simulink model "ctrl_student_HIL"  (R2015a)
settings: Solver=ode4  StartTime=0.0  StopTime=inf  FixedStep=0.01  RelTol=1e-3
(part 2 of 2)

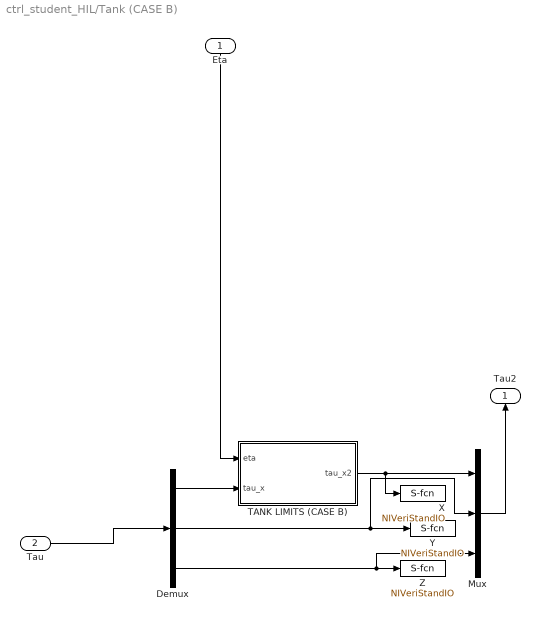
== system ctrl_student_HIL/Tank (CASE B) ==
  Eta : Inport
  Tau : Inport  Port=2
  Demux : Demux  Outputs=3
  Mux : Mux  Inputs=3
  TANK LIMITS (CASE B) : Subsystem
  X : S-Function  Priority=3  FunctionName=NIVeriStandIO  Parameters=width dtype portnum stime stype btype  mask(NI VeriStand Outport){portnum=3, width=-1, stime=-1, dtype=auto, stype=auto, btype=0}
      mask prompts: portnum "Port number:"; width "Port dimensions (-1 for dynamically sized):"; stime "Sample time (-1 for inherited):"; dtype "Data type:"; stype "Signal type:"; btype "Block type:"
      mask help: Use this outport on any level of nested subsystems to allow NI VeriStand software to map signals to it.
      mask init:
      | NIVeriStandIO_init;
      settings: CopyFcn=NIVeriStand_MDL_functions('', 'IO_copy');  DeleteFcn=NIVeriStand_MDL_functions('', 'IO_delete');  MoveFcn=set_param(gcb, 'Mask', 'on');
      mask Callback portnum: NIVeriStand_MDL_functions('', 'IO_setportnum');
      mask TypeOptions dtype: auto | double | single | int8 | uint8 | int16 | uint16 | int32 | uint32 | boolean
      mask Callback dtype: NIVeriStand_MDL_functions('', 'IO_booleansignal');
      mask TypeOptions stype: auto | real | complex
      mask Display:
      | patch([-x x], [-y y], [.90980 .81960 .32156]);
      | plot([xrad -x x xrad], [yrad -y y yrad]);
      | fprintf('NI Out%d', portnum);
  Y : S-Function  Priority=7  FunctionName=NIVeriStandIO  Parameters=width dtype portnum stime stype btype  mask(NI VeriStand Outport){portnum=7, width=-1, stime=-1, dtype=auto, stype=auto, btype=0}
      mask prompts: portnum "Port number:"; width "Port dimensions (-1 for dynamically sized):"; stime "Sample time (-1 for inherited):"; dtype "Data type:"; stype "Signal type:"; btype "Block type:"
      mask help: Use this outport on any level of nested subsystems to allow NI VeriStand software to map signals to it.
      mask init:
      | NIVeriStandIO_init;
      settings: CopyFcn=NIVeriStand_MDL_functions('', 'IO_copy');  DeleteFcn=NIVeriStand_MDL_functions('', 'IO_delete');  MoveFcn=set_param(gcb, 'Mask', 'on');
      mask Callback portnum: NIVeriStand_MDL_functions('', 'IO_setportnum');
      mask TypeOptions dtype: auto | double | single | int8 | uint8 | int16 | uint16 | int32 | uint32 | boolean
      mask Callback dtype: NIVeriStand_MDL_functions('', 'IO_booleansignal');
      mask TypeOptions stype: auto | real | complex
      mask Display:
      | patch([-x x], [-y y], [.90980 .81960 .32156]);
      | plot([xrad -x x xrad], [yrad -y y yrad]);
      | fprintf('NI Out%d', portnum);
  Z : S-Function  Priority=8  FunctionName=NIVeriStandIO  Parameters=width dtype portnum stime stype btype  mask(NI VeriStand Outport){portnum=8, width=-1, stime=-1, dtype=auto, stype=auto, btype=0}
      mask prompts: portnum "Port number:"; width "Port dimensions (-1 for dynamically sized):"; stime "Sample time (-1 for inherited):"; dtype "Data type:"; stype "Signal type:"; btype "Block type:"
      mask help: Use this outport on any level of nested subsystems to allow NI VeriStand software to map signals to it.
      mask init:
      | NIVeriStandIO_init;
      settings: CopyFcn=NIVeriStand_MDL_functions('', 'IO_copy');  DeleteFcn=NIVeriStand_MDL_functions('', 'IO_delete');  MoveFcn=set_param(gcb, 'Mask', 'on');
      mask Callback portnum: NIVeriStand_MDL_functions('', 'IO_setportnum');
      mask TypeOptions dtype: auto | double | single | int8 | uint8 | int16 | uint16 | int32 | uint32 | boolean
      mask Callback dtype: NIVeriStand_MDL_functions('', 'IO_booleansignal');
      mask TypeOptions stype: auto | real | complex
      mask Display:
      | patch([-x x], [-y y], [.90980 .81960 .32156]);
      | plot([xrad -x x xrad], [yrad -y y yrad]);
      | fprintf('NI Out%d', portnum);
  Tau2 : Outport
  wires:
  Mux/1 -> Tau2/1
  Tau/1 -> Demux/1
  TANK LIMITS (CASE B)/1(tau_x2) -> X/1, Mux/1
  Demux/1 -> TANK LIMITS (CASE B)/2(tau_x)
  Demux/2 -> Y/1, Mux/2
  Demux/3 -> Mux/3, Z/1
  Eta/1 -> TANK LIMITS (CASE B)/1(eta)

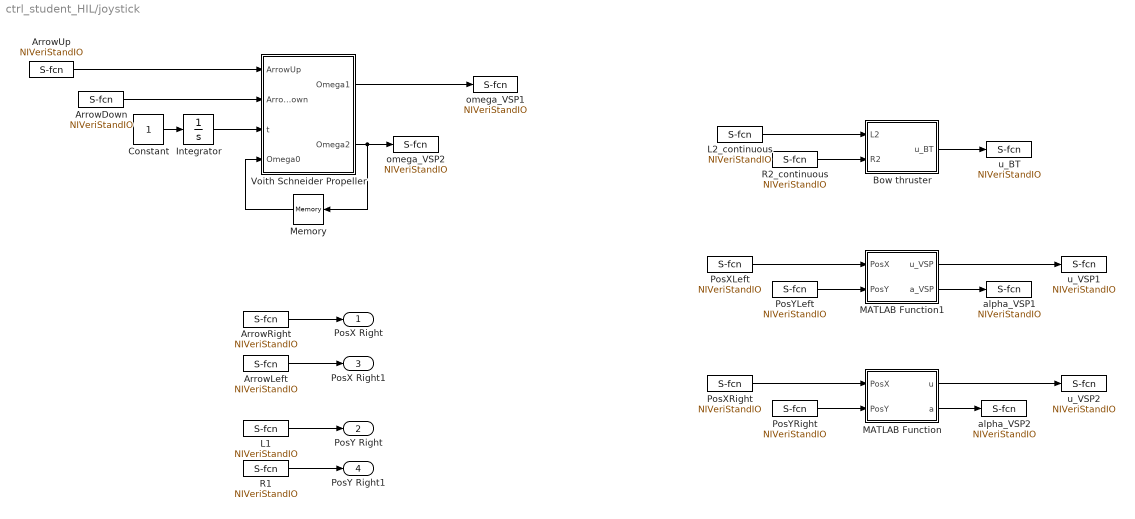
== system ctrl_student_HIL/joystick ==
  ArrowDown : S-Function  Priority=9  FunctionName=NIVeriStandIO  Parameters=width dtype portnum stime stype btype  mask(NI VeriStand Inport){portnum=9, width=-1, stime=-1, dtype=auto, stype=auto, btype=1}
      mask prompts: portnum "Port number:"; width "Port dimensions (-1 for dynamically sized):"; stime "Sample time (-1 for inherited):"; dtype "Data type:"; stype "Signal type:"; btype "Block type:"
      mask help: Use this inport on any level of nested subsystems to allow NI VeriStand software to map signals to it.
      mask init:
      | NIVeriStandIO_init;
      settings: CopyFcn=NIVeriStand_MDL_functions('', 'IO_copy');  DeleteFcn=NIVeriStand_MDL_functions('', 'IO_delete');  MoveFcn=set_param(gcb, 'Mask', 'on');
      mask Callback portnum: NIVeriStand_MDL_functions('', 'IO_setportnum');
      mask TypeOptions dtype: auto | double | single | int8 | uint8 | int16 | uint16 | int32 | uint32 | boolean
      mask Callback dtype: NIVeriStand_MDL_functions('', 'IO_booleansignal');
      mask TypeOptions stype: auto | real | complex
      mask Display:
      | patch([-x x], [-y y], [.90980 .81960 .32156]);
      | plot([xrad -x x xrad], [yrad -y y yrad]);
      | fprintf('NI In%d', portnum);
  ArrowLeft : S-Function  Priority=11  FunctionName=NIVeriStandIO  Parameters=width dtype portnum stime stype btype  mask(NI VeriStand Inport){portnum=11, width=-1, stime=-1, dtype=auto, stype=auto, btype=1}
      mask prompts: portnum "Port number:"; width "Port dimensions (-1 for dynamically sized):"; stime "Sample time (-1 for inherited):"; dtype "Data type:"; stype "Signal type:"; btype "Block type:"
      mask help: Use this inport on any level of nested subsystems to allow NI VeriStand software to map signals to it.
      mask init:
      | NIVeriStandIO_init;
      settings: CopyFcn=NIVeriStand_MDL_functions('', 'IO_copy');  DeleteFcn=NIVeriStand_MDL_functions('', 'IO_delete');  MoveFcn=set_param(gcb, 'Mask', 'on');
      mask Callback portnum: NIVeriStand_MDL_functions('', 'IO_setportnum');
      mask TypeOptions dtype: auto | double | single | int8 | uint8 | int16 | uint16 | int32 | uint32 | boolean
      mask Callback dtype: NIVeriStand_MDL_functions('', 'IO_booleansignal');
      mask TypeOptions stype: auto | real | complex
      mask Display:
      | patch([-x x], [-y y], [.90980 .81960 .32156]);
      | plot([xrad -x x xrad], [yrad -y y yrad]);
      | fprintf('NI In%d', portnum);
  ArrowRight : S-Function  Priority=12  FunctionName=NIVeriStandIO  Parameters=width dtype portnum stime stype btype  mask(NI VeriStand Inport){portnum=12, width=-1, stime=-1, dtype=auto, stype=auto, btype=1}
      mask prompts: portnum "Port number:"; width "Port dimensions (-1 for dynamically sized):"; stime "Sample time (-1 for inherited):"; dtype "Data type:"; stype "Signal type:"; btype "Block type:"
      mask help: Use this inport on any level of nested subsystems to allow NI VeriStand software to map signals to it.
      mask init:
      | NIVeriStandIO_init;
      settings: CopyFcn=NIVeriStand_MDL_functions('', 'IO_copy');  DeleteFcn=NIVeriStand_MDL_functions('', 'IO_delete');  MoveFcn=set_param(gcb, 'Mask', 'on');
      mask Callback portnum: NIVeriStand_MDL_functions('', 'IO_setportnum');
      mask TypeOptions dtype: auto | double | single | int8 | uint8 | int16 | uint16 | int32 | uint32 | boolean
      mask Callback dtype: NIVeriStand_MDL_functions('', 'IO_booleansignal');
      mask TypeOptions stype: auto | real | complex
      mask Display:
      | patch([-x x], [-y y], [.90980 .81960 .32156]);
      | plot([xrad -x x xrad], [yrad -y y yrad]);
      | fprintf('NI In%d', portnum);
  ArrowUp : S-Function  Priority=10  FunctionName=NIVeriStandIO  Parameters=width dtype portnum stime stype btype  mask(NI VeriStand Inport){portnum=10, width=-1, stime=-1, dtype=auto, stype=auto, btype=1}
      mask prompts: portnum "Port number:"; width "Port dimensions (-1 for dynamically sized):"; stime "Sample time (-1 for inherited):"; dtype "Data type:"; stype "Signal type:"; btype "Block type:"
      mask help: Use this inport on any level of nested subsystems to allow NI VeriStand software to map signals to it.
      mask init:
      | NIVeriStandIO_init;
      settings: CopyFcn=NIVeriStand_MDL_functions('', 'IO_copy');  DeleteFcn=NIVeriStand_MDL_functions('', 'IO_delete');  MoveFcn=set_param(gcb, 'Mask', 'on');
      mask Callback portnum: NIVeriStand_MDL_functions('', 'IO_setportnum');
      mask TypeOptions dtype: auto | double | single | int8 | uint8 | int16 | uint16 | int32 | uint32 | boolean
      mask Callback dtype: NIVeriStand_MDL_functions('', 'IO_booleansignal');
      mask TypeOptions stype: auto | real | complex
      mask Display:
      | patch([-x x], [-y y], [.90980 .81960 .32156]);
      | plot([xrad -x x xrad], [yrad -y y yrad]);
      | fprintf('NI In%d', portnum);
  Bow thruster : MATLAB Function  TreatAsAtomicUnit=on
  Constant : Constant
  Integrator : Integrator
  L1 : S-Function  Priority=7  FunctionName=NIVeriStandIO  Parameters=width dtype portnum stime stype btype  mask(NI VeriStand Inport){portnum=7, width=-1, stime=-1, dtype=auto, stype=auto, btype=1}
      mask prompts: portnum "Port number:"; width "Port dimensions (-1 for dynamically sized):"; stime "Sample time (-1 for inherited):"; dtype "Data type:"; stype "Signal type:"; btype "Block type:"
      mask help: Use this inport on any level of nested subsystems to allow NI VeriStand software to map signals to it.
      mask init:
      | NIVeriStandIO_init;
      settings: CopyFcn=NIVeriStand_MDL_functions('', 'IO_copy');  DeleteFcn=NIVeriStand_MDL_functions('', 'IO_delete');  MoveFcn=set_param(gcb, 'Mask', 'on');
      mask Callback portnum: NIVeriStand_MDL_functions('', 'IO_setportnum');
      mask TypeOptions dtype: auto | double | single | int8 | uint8 | int16 | uint16 | int32 | uint32 | boolean
      mask Callback dtype: NIVeriStand_MDL_functions('', 'IO_booleansignal');
      mask TypeOptions stype: auto | real | complex
      mask Display:
      | patch([-x x], [-y y], [.90980 .81960 .32156]);
      | plot([xrad -x x xrad], [yrad -y y yrad]);
      | fprintf('NI In%d', portnum);
  L2_continuous : S-Function  Priority=1  FunctionName=NIVeriStandIO  Parameters=width dtype portnum stime stype btype  mask(NI VeriStand Inport){portnum=1, width=-1, stime=-1, dtype=auto, stype=auto, btype=1}
      mask prompts: portnum "Port number:"; width "Port dimensions (-1 for dynamically sized):"; stime "Sample time (-1 for inherited):"; dtype "Data type:"; stype "Signal type:"; btype "Block type:"
      mask help: Use this inport on any level of nested subsystems to allow NI VeriStand software to map signals to it.
      mask init:
      | NIVeriStandIO_init;
      settings: CopyFcn=NIVeriStand_MDL_functions('', 'IO_copy');  DeleteFcn=NIVeriStand_MDL_functions('', 'IO_delete');  MoveFcn=set_param(gcb, 'Mask', 'on');
      mask Callback portnum: NIVeriStand_MDL_functions('', 'IO_setportnum');
      mask TypeOptions dtype: auto | double | single | int8 | uint8 | int16 | uint16 | int32 | uint32 | boolean
      mask Callback dtype: NIVeriStand_MDL_functions('', 'IO_booleansignal');
      mask TypeOptions stype: auto | real | complex
      mask Display:
      | patch([-x x], [-y y], [.90980 .81960 .32156]);
      | plot([xrad -x x xrad], [yrad -y y yrad]);
      | fprintf('NI In%d', portnum);
  MATLAB Function : MATLAB Function  TreatAsAtomicUnit=on
  MATLAB Function1 : MATLAB Function  TreatAsAtomicUnit=on
  Memory : Memory
  PosXLeft : S-Function  Priority=5  FunctionName=NIVeriStandIO  Parameters=width dtype portnum stime stype btype  mask(NI VeriStand Inport){portnum=5, width=-1, stime=-1, dtype=auto, stype=auto, btype=1}
      mask prompts: portnum "Port number:"; width "Port dimensions (-1 for dynamically sized):"; stime "Sample time (-1 for inherited):"; dtype "Data type:"; stype "Signal type:"; btype "Block type:"
      mask help: Use this inport on any level of nested subsystems to allow NI VeriStand software to map signals to it.
      mask init:
      | NIVeriStandIO_init;
      settings: CopyFcn=NIVeriStand_MDL_functions('', 'IO_copy');  DeleteFcn=NIVeriStand_MDL_functions('', 'IO_delete');  MoveFcn=set_param(gcb, 'Mask', 'on');
      mask Callback portnum: NIVeriStand_MDL_functions('', 'IO_setportnum');
      mask TypeOptions dtype: auto | double | single | int8 | uint8 | int16 | uint16 | int32 | uint32 | boolean
      mask Callback dtype: NIVeriStand_MDL_functions('', 'IO_booleansignal');
      mask TypeOptions stype: auto | real | complex
      mask Display:
      | patch([-x x], [-y y], [.90980 .81960 .32156]);
      | plot([xrad -x x xrad], [yrad -y y yrad]);
      | fprintf('NI In%d', portnum);
  PosXRight : S-Function  Priority=2  FunctionName=NIVeriStandIO  Parameters=width dtype portnum stime stype btype  mask(NI VeriStand Inport){portnum=2, width=-1, stime=-1, dtype=auto, stype=auto, btype=1}
      mask prompts: portnum "Port number:"; width "Port dimensions (-1 for dynamically sized):"; stime "Sample time (-1 for inherited):"; dtype "Data type:"; stype "Signal type:"; btype "Block type:"
      mask help: Use this inport on any level of nested subsystems to allow NI VeriStand software to map signals to it.
      mask init:
      | NIVeriStandIO_init;
      settings: CopyFcn=NIVeriStand_MDL_functions('', 'IO_copy');  DeleteFcn=NIVeriStand_MDL_functions('', 'IO_delete');  MoveFcn=set_param(gcb, 'Mask', 'on');
      mask Callback portnum: NIVeriStand_MDL_functions('', 'IO_setportnum');
      mask TypeOptions dtype: auto | double | single | int8 | uint8 | int16 | uint16 | int32 | uint32 | boolean
      mask Callback dtype: NIVeriStand_MDL_functions('', 'IO_booleansignal');
      mask TypeOptions stype: auto | real | complex
      mask Display:
      | patch([-x x], [-y y], [.90980 .81960 .32156]);
      | plot([xrad -x x xrad], [yrad -y y yrad]);
      | fprintf('NI In%d', portnum);
  PosYLeft : S-Function  Priority=6  FunctionName=NIVeriStandIO  Parameters=width dtype portnum stime stype btype  mask(NI VeriStand Inport){portnum=6, width=-1, stime=-1, dtype=auto, stype=auto, btype=1}
      mask prompts: portnum "Port number:"; width "Port dimensions (-1 for dynamically sized):"; stime "Sample time (-1 for inherited):"; dtype "Data type:"; stype "Signal type:"; btype "Block type:"
      mask help: Use this inport on any level of nested subsystems to allow NI VeriStand software to map signals to it.
      mask init:
      | NIVeriStandIO_init;
      settings: CopyFcn=NIVeriStand_MDL_functions('', 'IO_copy');  DeleteFcn=NIVeriStand_MDL_functions('', 'IO_delete');  MoveFcn=set_param(gcb, 'Mask', 'on');
      mask Callback portnum: NIVeriStand_MDL_functions('', 'IO_setportnum');
      mask TypeOptions dtype: auto | double | single | int8 | uint8 | int16 | uint16 | int32 | uint32 | boolean
      mask Callback dtype: NIVeriStand_MDL_functions('', 'IO_booleansignal');
      mask TypeOptions stype: auto | real | complex
      mask Display:
      | patch([-x x], [-y y], [.90980 .81960 .32156]);
      | plot([xrad -x x xrad], [yrad -y y yrad]);
      | fprintf('NI In%d', portnum);
  PosYRight : S-Function  Priority=3  FunctionName=NIVeriStandIO  Parameters=width dtype portnum stime stype btype  mask(NI VeriStand Inport){portnum=3, width=-1, stime=-1, dtype=auto, stype=auto, btype=1}
      mask prompts: portnum "Port number:"; width "Port dimensions (-1 for dynamically sized):"; stime "Sample time (-1 for inherited):"; dtype "Data type:"; stype "Signal type:"; btype "Block type:"
      mask help: Use this inport on any level of nested subsystems to allow NI VeriStand software to map signals to it.
      mask init:
      | NIVeriStandIO_init;
      settings: CopyFcn=NIVeriStand_MDL_functions('', 'IO_copy');  DeleteFcn=NIVeriStand_MDL_functions('', 'IO_delete');  MoveFcn=set_param(gcb, 'Mask', 'on');
      mask Callback portnum: NIVeriStand_MDL_functions('', 'IO_setportnum');
      mask TypeOptions dtype: auto | double | single | int8 | uint8 | int16 | uint16 | int32 | uint32 | boolean
      mask Callback dtype: NIVeriStand_MDL_functions('', 'IO_booleansignal');
      mask TypeOptions stype: auto | real | complex
      mask Display:
      | patch([-x x], [-y y], [.90980 .81960 .32156]);
      | plot([xrad -x x xrad], [yrad -y y yrad]);
      | fprintf('NI In%d', portnum);
  R1 : S-Function  Priority=8  FunctionName=NIVeriStandIO  Parameters=width dtype portnum stime stype btype  mask(NI VeriStand Inport){portnum=8, width=-1, stime=-1, dtype=auto, stype=auto, btype=1}
      mask prompts: portnum "Port number:"; width "Port dimensions (-1 for dynamically sized):"; stime "Sample time (-1 for inherited):"; dtype "Data type:"; stype "Signal type:"; btype "Block type:"
      mask help: Use this inport on any level of nested subsystems to allow NI VeriStand software to map signals to it.
      mask init:
      | NIVeriStandIO_init;
      settings: CopyFcn=NIVeriStand_MDL_functions('', 'IO_copy');  DeleteFcn=NIVeriStand_MDL_functions('', 'IO_delete');  MoveFcn=set_param(gcb, 'Mask', 'on');
      mask Callback portnum: NIVeriStand_MDL_functions('', 'IO_setportnum');
      mask TypeOptions dtype: auto | double | single | int8 | uint8 | int16 | uint16 | int32 | uint32 | boolean
      mask Callback dtype: NIVeriStand_MDL_functions('', 'IO_booleansignal');
      mask TypeOptions stype: auto | real | complex
      mask Display:
      | patch([-x x], [-y y], [.90980 .81960 .32156]);
      | plot([xrad -x x xrad], [yrad -y y yrad]);
      | fprintf('NI In%d', portnum);
  R2_continuous : S-Function  Priority=4  FunctionName=NIVeriStandIO  Parameters=width dtype portnum stime stype btype  mask(NI VeriStand Inport){portnum=4, width=-1, stime=-1, dtype=auto, stype=auto, btype=1}
      mask prompts: portnum "Port number:"; width "Port dimensions (-1 for dynamically sized):"; stime "Sample time (-1 for inherited):"; dtype "Data type:"; stype "Signal type:"; btype "Block type:"
      mask help: Use this inport on any level of nested subsystems to allow NI VeriStand software to map signals to it.
      mask init:
      | NIVeriStandIO_init;
      settings: CopyFcn=NIVeriStand_MDL_functions('', 'IO_copy');  DeleteFcn=NIVeriStand_MDL_functions('', 'IO_delete');  MoveFcn=set_param(gcb, 'Mask', 'on');
      mask Callback portnum: NIVeriStand_MDL_functions('', 'IO_setportnum');
      mask TypeOptions dtype: auto | double | single | int8 | uint8 | int16 | uint16 | int32 | uint32 | boolean
      mask Callback dtype: NIVeriStand_MDL_functions('', 'IO_booleansignal');
      mask TypeOptions stype: auto | real | complex
      mask Display:
      | patch([-x x], [-y y], [.90980 .81960 .32156]);
      | plot([xrad -x x xrad], [yrad -y y yrad]);
      | fprintf('NI In%d', portnum);
  Voith Schneider Propeller : MATLAB Function  TreatAsAtomicUnit=on
  alpha_VSP1 : S-Function  Priority=2  FunctionName=NIVeriStandIO  Parameters=width dtype portnum stime stype btype  mask(NI VeriStand Outport){portnum=2, width=-1, stime=-1, dtype=auto, stype=auto, btype=0}
      mask prompts: portnum "Port number:"; width "Port dimensions (-1 for dynamically sized):"; stime "Sample time (-1 for inherited):"; dtype "Data type:"; stype "Signal type:"; btype "Block type:"
      mask help: Use this outport on any level of nested subsystems to allow NI VeriStand software to map signals to it.
      mask init:
      | NIVeriStandIO_init;
      settings: CopyFcn=NIVeriStand_MDL_functions('', 'IO_copy');  DeleteFcn=NIVeriStand_MDL_functions('', 'IO_delete');  MoveFcn=set_param(gcb, 'Mask', 'on');
      mask Callback portnum: NIVeriStand_MDL_functions('', 'IO_setportnum');
      mask TypeOptions dtype: auto | double | single | int8 | uint8 | int16 | uint16 | int32 | uint32 | boolean
      mask Callback dtype: NIVeriStand_MDL_functions('', 'IO_booleansignal');
      mask TypeOptions stype: auto | real | complex
      mask Display:
      | patch([-x x], [-y y], [.90980 .81960 .32156]);
      | plot([xrad -x x xrad], [yrad -y y yrad]);
      | fprintf('NI Out%d', portnum);
  alpha_VSP2 : S-Function  Priority=6  FunctionName=NIVeriStandIO  Parameters=width dtype portnum stime stype btype  mask(NI VeriStand Outport){portnum=6, width=-1, stime=-1, dtype=auto, stype=auto, btype=0}
      mask prompts: portnum "Port number:"; width "Port dimensions (-1 for dynamically sized):"; stime "Sample time (-1 for inherited):"; dtype "Data type:"; stype "Signal type:"; btype "Block type:"
      mask help: Use this outport on any level of nested subsystems to allow NI VeriStand software to map signals to it.
      mask init:
      | NIVeriStandIO_init;
      settings: CopyFcn=NIVeriStand_MDL_functions('', 'IO_copy');  DeleteFcn=NIVeriStand_MDL_functions('', 'IO_delete');  MoveFcn=set_param(gcb, 'Mask', 'on');
      mask Callback portnum: NIVeriStand_MDL_functions('', 'IO_setportnum');
      mask TypeOptions dtype: auto | double | single | int8 | uint8 | int16 | uint16 | int32 | uint32 | boolean
      mask Callback dtype: NIVeriStand_MDL_functions('', 'IO_booleansignal');
      mask TypeOptions stype: auto | real | complex
      mask Display:
      | patch([-x x], [-y y], [.90980 .81960 .32156]);
      | plot([xrad -x x xrad], [yrad -y y yrad]);
      | fprintf('NI Out%d', portnum);
  omega_VSP1 : S-Function  Priority=3  FunctionName=NIVeriStandIO  Parameters=width dtype portnum stime stype btype  mask(NI VeriStand Outport){portnum=3, width=-1, stime=-1, dtype=auto, stype=auto, btype=0}
      mask prompts: portnum "Port number:"; width "Port dimensions (-1 for dynamically sized):"; stime "Sample time (-1 for inherited):"; dtype "Data type:"; stype "Signal type:"; btype "Block type:"
      mask help: Use this outport on any level of nested subsystems to allow NI VeriStand software to map signals to it.
      mask init:
      | NIVeriStandIO_init;
      settings: CopyFcn=NIVeriStand_MDL_functions('', 'IO_copy');  DeleteFcn=NIVeriStand_MDL_functions('', 'IO_delete');  MoveFcn=set_param(gcb, 'Mask', 'on');
      mask Callback portnum: NIVeriStand_MDL_functions('', 'IO_setportnum');
      mask TypeOptions dtype: auto | double | single | int8 | uint8 | int16 | uint16 | int32 | uint32 | boolean
      mask Callback dtype: NIVeriStand_MDL_functions('', 'IO_booleansignal');
      mask TypeOptions stype: auto | real | complex
      mask Display:
      | patch([-x x], [-y y], [.90980 .81960 .32156]);
      | plot([xrad -x x xrad], [yrad -y y yrad]);
      | fprintf('NI Out%d', portnum);
  omega_VSP2 : S-Function  Priority=4  FunctionName=NIVeriStandIO  Parameters=width dtype portnum stime stype btype  mask(NI VeriStand Outport){portnum=4, width=-1, stime=-1, dtype=auto, stype=auto, btype=0}
      mask prompts: portnum "Port number:"; width "Port dimensions (-1 for dynamically sized):"; stime "Sample time (-1 for inherited):"; dtype "Data type:"; stype "Signal type:"; btype "Block type:"
      mask help: Use this outport on any level of nested subsystems to allow NI VeriStand software to map signals to it.
      mask init:
      | NIVeriStandIO_init;
      settings: CopyFcn=NIVeriStand_MDL_functions('', 'IO_copy');  DeleteFcn=NIVeriStand_MDL_functions('', 'IO_delete');  MoveFcn=set_param(gcb, 'Mask', 'on');
      mask Callback portnum: NIVeriStand_MDL_functions('', 'IO_setportnum');
      mask TypeOptions dtype: auto | double | single | int8 | uint8 | int16 | uint16 | int32 | uint32 | boolean
      mask Callback dtype: NIVeriStand_MDL_functions('', 'IO_booleansignal');
      mask TypeOptions stype: auto | real | complex
      mask Display:
      | patch([-x x], [-y y], [.90980 .81960 .32156]);
      | plot([xrad -x x xrad], [yrad -y y yrad]);
      | fprintf('NI Out%d', portnum);
  u_BT : S-Function  Priority=5  FunctionName=NIVeriStandIO  Parameters=width dtype portnum stime stype btype  mask(NI VeriStand Outport){portnum=5, width=-1, stime=-1, dtype=auto, stype=auto, btype=0}
      mask prompts: portnum "Port number:"; width "Port dimensions (-1 for dynamically sized):"; stime "Sample time (-1 for inherited):"; dtype "Data type:"; stype "Signal type:"; btype "Block type:"
      mask help: Use this outport on any level of nested subsystems to allow NI VeriStand software to map signals to it.
      mask init:
      | NIVeriStandIO_init;
      settings: CopyFcn=NIVeriStand_MDL_functions('', 'IO_copy');  DeleteFcn=NIVeriStand_MDL_functions('', 'IO_delete');  MoveFcn=set_param(gcb, 'Mask', 'on');
      mask Callback portnum: NIVeriStand_MDL_functions('', 'IO_setportnum');
      mask TypeOptions dtype: auto | double | single | int8 | uint8 | int16 | uint16 | int32 | uint32 | boolean
      mask Callback dtype: NIVeriStand_MDL_functions('', 'IO_booleansignal');
      mask TypeOptions stype: auto | real | complex
      mask Display:
      | patch([-x x], [-y y], [.90980 .81960 .32156]);
      | plot([xrad -x x xrad], [yrad -y y yrad]);
      | fprintf('NI Out%d', portnum);
  u_VSP1 : S-Function  Priority=1  FunctionName=NIVeriStandIO  Parameters=width dtype portnum stime stype btype  mask(NI VeriStand Outport){portnum=1, width=-1, stime=-1, dtype=auto, stype=auto, btype=0}
      mask prompts: portnum "Port number:"; width "Port dimensions (-1 for dynamically sized):"; stime "Sample time (-1 for inherited):"; dtype "Data type:"; stype "Signal type:"; btype "Block type:"
      mask help: Use this outport on any level of nested subsystems to allow NI VeriStand software to map signals to it.
      mask init:
      | NIVeriStandIO_init;
      settings: CopyFcn=NIVeriStand_MDL_functions('', 'IO_copy');  DeleteFcn=NIVeriStand_MDL_functions('', 'IO_delete');  MoveFcn=set_param(gcb, 'Mask', 'on');
      mask Callback portnum: NIVeriStand_MDL_functions('', 'IO_setportnum');
      mask TypeOptions dtype: auto | double | single | int8 | uint8 | int16 | uint16 | int32 | uint32 | boolean
      mask Callback dtype: NIVeriStand_MDL_functions('', 'IO_booleansignal');
      mask TypeOptions stype: auto | real | complex
      mask Display:
      | patch([-x x], [-y y], [.90980 .81960 .32156]);
      | plot([xrad -x x xrad], [yrad -y y yrad]);
      | fprintf('NI Out%d', portnum);
  u_VSP2 : S-Function  Priority=7  FunctionName=NIVeriStandIO  Parameters=width dtype portnum stime stype btype  mask(NI VeriStand Outport){portnum=7, width=-1, stime=-1, dtype=auto, stype=auto, btype=0}
      mask prompts: portnum "Port number:"; width "Port dimensions (-1 for dynamically sized):"; stime "Sample time (-1 for inherited):"; dtype "Data type:"; stype "Signal type:"; btype "Block type:"
      mask help: Use this outport on any level of nested subsystems to allow NI VeriStand software to map signals to it.
      mask init:
      | NIVeriStandIO_init;
      settings: CopyFcn=NIVeriStand_MDL_functions('', 'IO_copy');  DeleteFcn=NIVeriStand_MDL_functions('', 'IO_delete');  MoveFcn=set_param(gcb, 'Mask', 'on');
      mask Callback portnum: NIVeriStand_MDL_functions('', 'IO_setportnum');
      mask TypeOptions dtype: auto | double | single | int8 | uint8 | int16 | uint16 | int32 | uint32 | boolean
      mask Callback dtype: NIVeriStand_MDL_functions('', 'IO_booleansignal');
      mask TypeOptions stype: auto | real | complex
      mask Display:
      | patch([-x x], [-y y], [.90980 .81960 .32156]);
      | plot([xrad -x x xrad], [yrad -y y yrad]);
      | fprintf('NI Out%d', portnum);
  PosX Right : Outport
  PosY Right : Outport  Port=2
  PosX Right1 : Outport  Port=3
  PosY Right1 : Outport  Port=4
  wires:
  L2_continuous/1 -> Bow thruster/1(L2)
  Voith Schneider Propeller/2(Omega2) -> omega_VSP2/1, Memory/1
  Voith Schneider Propeller/1(Omega1) -> omega_VSP1/1
  PosXRight/1 -> MATLAB Function/1(PosX)
  MATLAB Function/1(u) -> u_VSP2/1
  PosYRight/1 -> MATLAB Function/2(PosY)
  MATLAB Function/2(a) -> alpha_VSP2/1
  PosXLeft/1 -> MATLAB Function1/1(PosX)
  MATLAB Function1/1(u_VSP) -> u_VSP1/1
  PosYLeft/1 -> MATLAB Function1/2(PosY)
  MATLAB Function1/2(a_VSP) -> alpha_VSP1/1
  Constant/1 -> Integrator/1
  Memory/1 -> Voith Schneider Propeller/4(Omega0)
  Integrator/1 -> Voith Schneider Propeller/3(t)
  ArrowDown/1 -> Voith Schneider Propeller/2(ArrowDown)
  ArrowUp/1 -> Voith Schneider Propeller/1(ArrowUp)
  R2_continuous/1 -> Bow thruster/2(R2)
  Bow thruster/1(u_BT) -> u_BT/1
  R1/1 -> PosY Right1/1
  L1/1 -> PosY Right/1
  ArrowRight/1 -> PosX Right/1
  ArrowLeft/1 -> PosX Right1/1

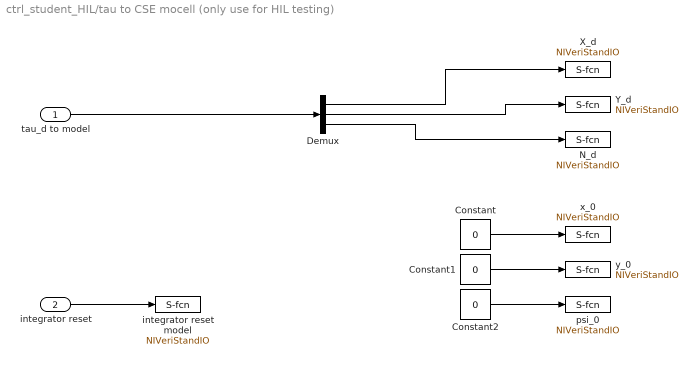
== system ctrl_student_HIL/tau to CSE mocell (only use for HIL testing) ==
  tau_d to model : Inport
  integrator reset : Inport  Port=2
  Constant : Constant  Value=0
  Constant1 : Constant  Value=0
  Constant2 : Constant  Value=0
  Demux : Demux  Outputs=3
  N_d : S-Function  Priority=2  FunctionName=NIVeriStandIO  Parameters=width dtype portnum stime stype btype  mask(NI VeriStand Outport){portnum=2, width=-1, stime=-1, dtype=auto, stype=auto, btype=0}
      mask prompts: portnum "Port number:"; width "Port dimensions (-1 for dynamically sized):"; stime "Sample time (-1 for inherited):"; dtype "Data type:"; stype "Signal type:"; btype "Block type:"
      mask help: Use this outport on any level of nested subsystems to allow NI VeriStand software to map signals to it.
      mask init:
      | NIVeriStandIO_init;
      settings: CopyFcn=NIVeriStand_MDL_functions('', 'IO_copy');  DeleteFcn=NIVeriStand_MDL_functions('', 'IO_delete');  MoveFcn=set_param(gcb, 'Mask', 'on');
      mask Callback portnum: NIVeriStand_MDL_functions('', 'IO_setportnum');
      mask TypeOptions dtype: auto | double | single | int8 | uint8 | int16 | uint16 | int32 | uint32 | boolean
      mask Callback dtype: NIVeriStand_MDL_functions('', 'IO_booleansignal');
      mask TypeOptions stype: auto | real | complex
      mask Display:
      | patch([-x x], [-y y], [.90980 .81960 .32156]);
      | plot([xrad -x x xrad], [yrad -y y yrad]);
      | fprintf('NI Out%d', portnum);
  X_d : S-Function  Priority=1  FunctionName=NIVeriStandIO  Parameters=width dtype portnum stime stype btype  mask(NI VeriStand Outport){portnum=1, width=-1, stime=-1, dtype=auto, stype=auto, btype=0}
      mask prompts: portnum "Port number:"; width "Port dimensions (-1 for dynamically sized):"; stime "Sample time (-1 for inherited):"; dtype "Data type:"; stype "Signal type:"; btype "Block type:"
      mask help: Use this outport on any level of nested subsystems to allow NI VeriStand software to map signals to it.
      mask init:
      | NIVeriStandIO_init;
      settings: CopyFcn=NIVeriStand_MDL_functions('', 'IO_copy');  DeleteFcn=NIVeriStand_MDL_functions('', 'IO_delete');  MoveFcn=set_param(gcb, 'Mask', 'on');
      mask Callback portnum: NIVeriStand_MDL_functions('', 'IO_setportnum');
      mask TypeOptions dtype: auto | double | single | int8 | uint8 | int16 | uint16 | int32 | uint32 | boolean
      mask Callback dtype: NIVeriStand_MDL_functions('', 'IO_booleansignal');
      mask TypeOptions stype: auto | real | complex
      mask Display:
      | patch([-x x], [-y y], [.90980 .81960 .32156]);
      | plot([xrad -x x xrad], [yrad -y y yrad]);
      | fprintf('NI Out%d', portnum);
  Y_d : S-Function  Priority=3  FunctionName=NIVeriStandIO  Parameters=width dtype portnum stime stype btype  mask(NI VeriStand Outport){portnum=3, width=-1, stime=-1, dtype=auto, stype=auto, btype=0}
      mask prompts: portnum "Port number:"; width "Port dimensions (-1 for dynamically sized):"; stime "Sample time (-1 for inherited):"; dtype "Data type:"; stype "Signal type:"; btype "Block type:"
      mask help: Use this outport on any level of nested subsystems to allow NI VeriStand software to map signals to it.
      mask init:
      | NIVeriStandIO_init;
      settings: CopyFcn=NIVeriStand_MDL_functions('', 'IO_copy');  DeleteFcn=NIVeriStand_MDL_functions('', 'IO_delete');  MoveFcn=set_param(gcb, 'Mask', 'on');
      mask Callback portnum: NIVeriStand_MDL_functions('', 'IO_setportnum');
      mask TypeOptions dtype: auto | double | single | int8 | uint8 | int16 | uint16 | int32 | uint32 | boolean
      mask Callback dtype: NIVeriStand_MDL_functions('', 'IO_booleansignal');
      mask TypeOptions stype: auto | real | complex
      mask Display:
      | patch([-x x], [-y y], [.90980 .81960 .32156]);
      | plot([xrad -x x xrad], [yrad -y y yrad]);
      | fprintf('NI Out%d', portnum);
  integrator reset model : S-Function  Priority=7  FunctionName=NIVeriStandIO  Parameters=width dtype portnum stime stype btype  mask(NI VeriStand Outport){portnum=7, width=-1, stime=-1, dtype=auto, stype=auto, btype=0}
      mask prompts: portnum "Port number:"; width "Port dimensions (-1 for dynamically sized):"; stime "Sample time (-1 for inherited):"; dtype "Data type:"; stype "Signal type:"; btype "Block type:"
      mask help: Use this outport on any level of nested subsystems to allow NI VeriStand software to map signals to it.
      mask init:
      | NIVeriStandIO_init;
      settings: CopyFcn=NIVeriStand_MDL_functions('', 'IO_copy');  DeleteFcn=NIVeriStand_MDL_functions('', 'IO_delete');  MoveFcn=set_param(gcb, 'Mask', 'on');
      mask Callback portnum: NIVeriStand_MDL_functions('', 'IO_setportnum');
      mask TypeOptions dtype: auto | double | single | int8 | uint8 | int16 | uint16 | int32 | uint32 | boolean
      mask Callback dtype: NIVeriStand_MDL_functions('', 'IO_booleansignal');
      mask TypeOptions stype: auto | real | complex
      mask Display:
      | patch([-x x], [-y y], [.90980 .81960 .32156]);
      | plot([xrad -x x xrad], [yrad -y y yrad]);
      | fprintf('NI Out%d', portnum);
  "psi_0 " : S-Function  Priority=4  FunctionName=NIVeriStandIO  Parameters=width dtype portnum stime stype btype  mask(NI VeriStand Outport){portnum=4, width=-1, stime=-1, dtype=auto, stype=auto, btype=0}
      mask prompts: portnum "Port number:"; width "Port dimensions (-1 for dynamically sized):"; stime "Sample time (-1 for inherited):"; dtype "Data type:"; stype "Signal type:"; btype "Block type:"
      mask help: Use this outport on any level of nested subsystems to allow NI VeriStand software to map signals to it.
      mask init:
      | NIVeriStandIO_init;
      settings: CopyFcn=NIVeriStand_MDL_functions('', 'IO_copy');  DeleteFcn=NIVeriStand_MDL_functions('', 'IO_delete');  MoveFcn=set_param(gcb, 'Mask', 'on');
      mask Callback portnum: NIVeriStand_MDL_functions('', 'IO_setportnum');
      mask TypeOptions dtype: auto | double | single | int8 | uint8 | int16 | uint16 | int32 | uint32 | boolean
      mask Callback dtype: NIVeriStand_MDL_functions('', 'IO_booleansignal');
      mask TypeOptions stype: auto | real | complex
      mask Display:
      | patch([-x x], [-y y], [.90980 .81960 .32156]);
      | plot([xrad -x x xrad], [yrad -y y yrad]);
      | fprintf('NI Out%d', portnum);
  x_0 : S-Function  Priority=5  FunctionName=NIVeriStandIO  Parameters=width dtype portnum stime stype btype  mask(NI VeriStand Outport){portnum=5, width=-1, stime=-1, dtype=auto, stype=auto, btype=0}
      mask prompts: portnum "Port number:"; width "Port dimensions (-1 for dynamically sized):"; stime "Sample time (-1 for inherited):"; dtype "Data type:"; stype "Signal type:"; btype "Block type:"
      mask help: Use this outport on any level of nested subsystems to allow NI VeriStand software to map signals to it.
      mask init:
      | NIVeriStandIO_init;
      settings: CopyFcn=NIVeriStand_MDL_functions('', 'IO_copy');  DeleteFcn=NIVeriStand_MDL_functions('', 'IO_delete');  MoveFcn=set_param(gcb, 'Mask', 'on');
      mask Callback portnum: NIVeriStand_MDL_functions('', 'IO_setportnum');
      mask TypeOptions dtype: auto | double | single | int8 | uint8 | int16 | uint16 | int32 | uint32 | boolean
      mask Callback dtype: NIVeriStand_MDL_functions('', 'IO_booleansignal');
      mask TypeOptions stype: auto | real | complex
      mask Display:
      | patch([-x x], [-y y], [.90980 .81960 .32156]);
      | plot([xrad -x x xrad], [yrad -y y yrad]);
      | fprintf('NI Out%d', portnum);
  y_0 : S-Function  Priority=6  FunctionName=NIVeriStandIO  Parameters=width dtype portnum stime stype btype  mask(NI VeriStand Outport){portnum=6, width=-1, stime=-1, dtype=auto, stype=auto, btype=0}
      mask prompts: portnum "Port number:"; width "Port dimensions (-1 for dynamically sized):"; stime "Sample time (-1 for inherited):"; dtype "Data type:"; stype "Signal type:"; btype "Block type:"
      mask help: Use this outport on any level of nested subsystems to allow NI VeriStand software to map signals to it.
      mask init:
      | NIVeriStandIO_init;
      settings: CopyFcn=NIVeriStand_MDL_functions('', 'IO_copy');  DeleteFcn=NIVeriStand_MDL_functions('', 'IO_delete');  MoveFcn=set_param(gcb, 'Mask', 'on');
      mask Callback portnum: NIVeriStand_MDL_functions('', 'IO_setportnum');
      mask TypeOptions dtype: auto | double | single | int8 | uint8 | int16 | uint16 | int32 | uint32 | boolean
      mask Callback dtype: NIVeriStand_MDL_functions('', 'IO_booleansignal');
      mask TypeOptions stype: auto | real | complex
      mask Display:
      | patch([-x x], [-y y], [.90980 .81960 .32156]);
      | plot([xrad -x x xrad], [yrad -y y yrad]);
      | fprintf('NI Out%d', portnum);
  wires:
  tau_d to model/1 -> Demux/1
  Demux/1 -> X_d/1
  Demux/2 -> Y_d/1
  Demux/3 -> N_d/1
  Constant2/1 -> "psi_0 "/1
  Constant1/1 -> y_0/1
  Constant/1 -> x_0/1
  integrator reset/1 -> integrator reset model/1

== system ctrl_student_HIL/Noise generator/Downsample	signal ==
  sampling frequency : Inport
  step size : Inport  Port=2
  MATLAB Function : MATLAB Function  TreatAsAtomicUnit=on
  counter : Memory
  trigger : Outport
  wires:
  sampling frequency/1 -> MATLAB Function/1(f)
  step size/1 -> MATLAB Function/2(h)
  counter/1 -> MATLAB Function/3(i)
  MATLAB Function/1(count) -> counter/1, trigger/1

== system ctrl_student_HIL/Noise generator/Sample & hold ==
  trigger : Inport
  input : Inport  Port=2
  Hold : Memory
  MATLAB Function1 : MATLAB Function  TreatAsAtomicUnit=on
  output : Outport
  wires:
  MATLAB Function1/1(output) -> output/1, Hold/1
  trigger/1 -> MATLAB Function1/1(counter)
  input/1 -> MATLAB Function1/2(input)
  Hold/1 -> MATLAB Function1/3(hold)

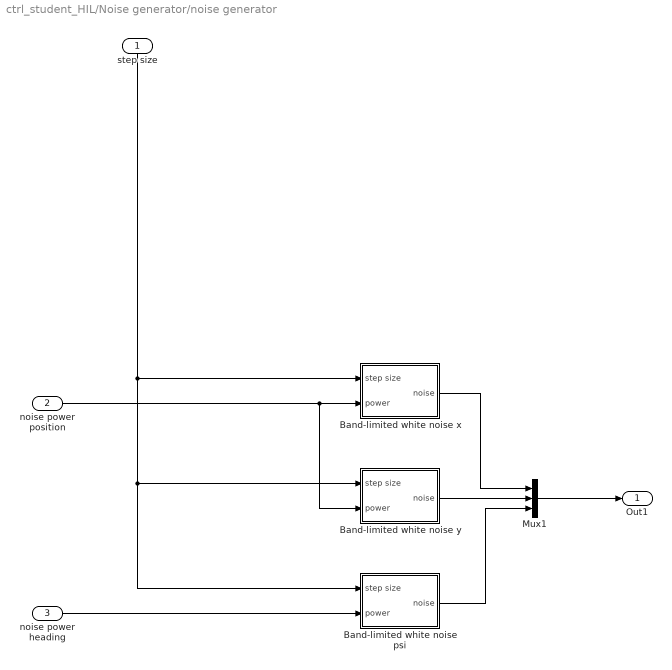
== system ctrl_student_HIL/Noise generator/noise generator ==
  step size : Inport
  noise power position : Inport  Port=2
  noise power heading : Inport  Port=3
  Band-limited white noise psi : Subsystem
  Band-limited white noise x : Subsystem
  Band-limited white noise y : Subsystem
  Mux1 : Mux  Inputs=3
  Out1 : Outport
  wires:
  Mux1/1 -> Out1/1
  step size/1 -> Band-limited white noise x/1(step size), Band-limited white noise psi/1(step size), Band-limited white noise y/1(step size)
  noise power position/1 -> Band-limited white noise y/2(power), Band-limited white noise x/2(power)
  Band-limited white noise x/1(noise) -> Mux1/1
  Band-limited white noise y/1(noise) -> Mux1/2
  Band-limited white noise psi/1(noise) -> Mux1/3
  noise power heading/1 -> Band-limited white noise psi/2(power)

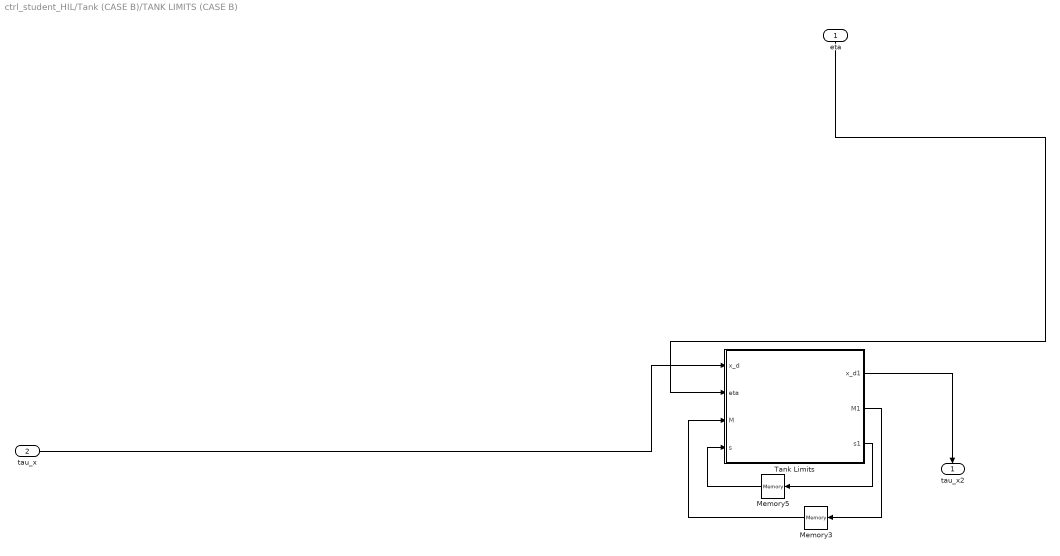
== system ctrl_student_HIL/Tank (CASE B)/TANK LIMITS (CASE B) ==
  eta : Inport
  tau_x : Inport  Port=2
  Memory3 : Memory
  Memory5 : Memory  X0=1
  Tank Limits : MATLAB Function  TreatAsAtomicUnit=on
  tau_x2 : Outport
  wires:
  Tank Limits/1(x_d1) -> tau_x2/1
  Tank Limits/3(s1) -> Memory5/1
  tau_x/1 -> Tank Limits/1(x_d)
  Tank Limits/2(M1) -> Memory3/1
  Memory3/1 -> Tank Limits/3(M)
  Memory5/1 -> Tank Limits/4(s)
  eta/1 -> Tank Limits/2(eta)

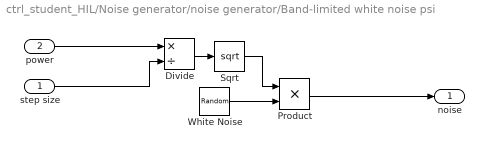
== system ctrl_student_HIL/Noise generator/noise generator/Band-limited white noise psi ==
  step size : Inport
  power : Inport  Port=2
  Divide : Product  Inputs=*/
  Product : Product
  Sqrt : Sqrt  SaturateOnIntegerOverflow=on
  White Noise : RandomNumber  DisableCoverage=on  Seed=9025
  noise : Outport
  wires:
  White Noise/1 -> Product/2
  Product/1 -> noise/1
  step size/1 -> Divide/2
  Divide/1 -> Sqrt/1
  Sqrt/1 -> Product/1
  power/1 -> Divide/1

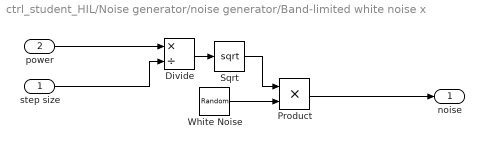
== system ctrl_student_HIL/Noise generator/noise generator/Band-limited white noise x ==
  step size : Inport
  power : Inport  Port=2
  Divide : Product  Inputs=*/
  Product : Product
  Sqrt : Sqrt  SaturateOnIntegerOverflow=on
  White Noise : RandomNumber  DisableCoverage=on  Seed=9024
  noise : Outport
  wires:
  White Noise/1 -> Product/2
  Product/1 -> noise/1
  step size/1 -> Divide/2
  Divide/1 -> Sqrt/1
  Sqrt/1 -> Product/1
  power/1 -> Divide/1

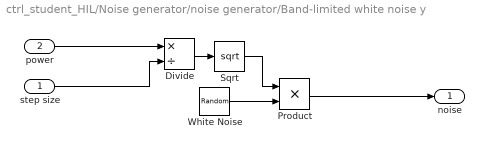
== system ctrl_student_HIL/Noise generator/noise generator/Band-limited white noise y ==
  step size : Inport
  power : Inport  Port=2
  Divide : Product  Inputs=*/
  Product : Product
  Sqrt : Sqrt  SaturateOnIntegerOverflow=on
  White Noise : RandomNumber  DisableCoverage=on  Seed=123
  noise : Outport
  wires:
  White Noise/1 -> Product/2
  Product/1 -> noise/1
  step size/1 -> Divide/2
  Divide/1 -> Sqrt/1
  Sqrt/1 -> Product/1
  power/1 -> Divide/1

== matlab function ctrl_student_HIL/Guidance (CASE D)/Control Law ==
  data: k2 input; s_dot input; Us input; Us_s input; eta_d input; eta_ds input; eta_ds2 input; eta input; Tau output; Rz1 output; nu input
function [Tau,Rz1] = fcn(k2,s_dot,Us,Us_s,eta_d,eta_ds,eta_ds2,eta,nu)

%% ROTATION MATRICES

psi = 0;
Tau = [0;0;0];
psi = eta(3);   % psi : yaw angle
r = nu(3);      % r : yaw rate
u = nu(1);      % u : surge velocity
v = nu(2);      % v : sway velocity


R = [ cos(psi) , -sin(psi) , 0 ;
      sin(psi) , cos(psi)  , 0 ;
      0            0         1 ] ;

S = [ 0 , -r , 0 ;
       r , 0 , 0 ;
       0 , 0 , 0 ];

   
%% MASS MATRIX (from CSEI_tau)

m    = 14.79;   I_z  =  1.7600;   x_g = 0.0375;       % x_g  =  0.0460; % Table B.1

% Added mass
X_ud  =     -2.0;											% Table B.1
					Y_vd =     -1.0;	N_vd =    -0.0;		% Table B.1 guestimate
					Y_rd =      -0.0;	N_rd =    -1.0;		% Table B.1
                    
% Total mass matrix
m_11 = m-X_ud;
m_22 = m-Y_vd;
m_23 = m*x_g-Y_rd;
m_32 = m*x_g-N_vd;
m_33 = I_z-N_rd;

M    = [m_11 0    0
        0    m_22 m_23
        0    m_32 m_33];
	
%% DAMPING MATRIX (from CSEI_tau)
X_u		= -0.6555;		X_v		= 0;
X_uu 	= 0.3545;		X_vv	= -2.443;
X_uuu 	= -3.787;		X_vvv	= 0;

						Y_v		= -1.33; 			Y_r		= -7.250; % Y_r
						Y_vv	= -2.776;			Y_rr	= -3.450; % Y_rr
						Y_vvv	= -64.91;			Y_rrr	= 0;
						
						Y_rv	= -0.805;			Y_vr	= -0.845; % Y_rv, Y_vr

						N_v		= 0;				N_r		= -1.900; % N_r
						N_vv	= -0.2088;			N_rr	= -0.750; % N_rr
						N_vvv	= 0;				N_rrr	= 0;
						
						N_rv	= 0.130;			N_vr	= 0.080; % N_rv, N_vr

% Assembly of the damping matrix
d_11 = -X_u - X_uu*u - X_uuu*u^2;
d_22 = -Y_v - Y_vv*v - Y_vvv*v^2 - Y_rv*abs(r);
d_33 = -N_r - N_rr*abs(r) - N_rrr*r^2 - N_vr*abs(v); % using abs(r)

d_12 = -X_v - X_vv*v - X_vvv*v^2;
d_23 = -Y_r - Y_rr*abs(r) - Y_rrr*r^2 - Y_vr*abs(v);
d_32 = -N_v - N_vv*v - N_vvv*v^2 - N_rv*abs(r);

D    = [d_11 0 0
        0    d_22 d_23
        0    d_32 d_33];


%% CASE D


K_p = diag([0.2,0.2,0.1]);          % Kp (tuning)
K2 = k2 * diag([1,1,1]);           % K2 (tuning)

z1 = R'*(eta-eta_d);                % z1
alpha1 = -K_p*z1 + R'*eta_ds*Us ;   % alpha1
Rz1 = R*z1 ;                        % R*z1

z1_dot = S'*z1+nu-R'*eta_ds*s_dot;  % z1_dot
a1_dot = -K_p*z1_dot+(R*S)'*eta_ds*Us + R'*(eta_ds2*Us+eta_ds*Us_s)*s_dot;    % alpha1_dot

z2 = nu - alpha1 ;                  % z2

Tau = D*nu  +   M*a1_dot - K2*z2 - z1 ;     % Tau



end

== matlab function ctrl_student_HIL/Guidance (CASE D)/Guidance (Ellipse) ==
  data: s input; s_dot output; Us output; U_ref1 input; mu input; Rz1 input; Us_s output; eta_d output; eta_ds output; eta_ds2 output
function [s_dot,Us,Us_s,eta_d,eta_ds,eta_ds2] = f(s,U_ref1,mu,Rz1)

%% Ellipse Kinematics

eta_d = [0;0;0];
eta_ds = [0;0;0];
eta_ds2 = [0;0;0];

cx = 6;
cy = 0;
rx = 5;
ry = 3;

x_d = cx+rx*cos(s);
y_d = cy+ry*sin(s);

x_ds = -rx*sin(s);
y_ds = ry*cos(s);

x_ds2 = -rx*cos(s);
y_ds2 = -ry*sin(s);

x_ds3 = rx*sin(s);
y_ds3 = -ry*cos(s);

psi_d = atan2(y_ds,x_ds);
psi_ds = (-y_ds*x_ds+x_ds*y_ds2)/(x_ds^2+y_ds^2);
psi_ds2 = ( (-y_ds*x_ds3+x_ds*y_ds3)*(x_ds^2+y_ds^2) - (-y_ds*x_ds2+x_ds*y_ds2)*(2*x_ds2*x_ds+2*y_ds2*y_ds) )/(x_ds^2+y_ds^2)^2;

eta_d = [x_d;y_d;psi_d] ;
eta_ds = [x_ds;y_ds;psi_ds];
eta_ds2 = [x_ds2;y_ds2;psi_ds2];

Us = U_ref1 / (x_ds^2+y_ds^2)^(1/2);
Us_s = U_ref1 * (x_ds*x_ds2 + y_ds*y_ds2) / (x_ds^2+y_ds^2)^(3/2);


%% Update Law

V1 = - eta_ds'*Rz1 ;
s_dot = Us - mu*V1/norm(eta_ds);


end

== matlab function ctrl_student_HIL/Observer (CASE C)/DP Observer ==
  data: eta_m input; L1_o input; L2_o input; L3_o input; Tau input; x input; x_dot output
function x_dot = fcn(eta_m,L1_o,L2_o,L3_o,Tau,x)
%#codegen

%% INPUT PARAMETERS

m = 14.79 ;

M = [ m + 2 , 0     ,   0          ;
      0  ,   m + 10, m*0.0375      ;
      0  , m*0.0375 ,   1.76 + 1 ] ;     % Mass matrix
  
u = x(4);       % Surge velocity
v = x(5);       % Sway velocity
r = x(6);       % Yaw rate
psi = eta_m(3); % Heading
Inv = inv(M) ;  % Inverse of M

X_u = - 0.6555 ;
X_uu = 0.3545 ;
X_uuu = - 3.787 ;
Y_v = - 1.33 ;
Y_vv = -2.776  ;
Y_vvv = -64.91 ;
Y_r = -7.25 ;
Y_rr = - 3.45 ;
Y_rrr = 0;
Y_vr = -0.845 ;
Y_rv = -0.805 ;
N_v = 0 ;
N_vv = - 0.2088 ;
N_vvv = 0;
N_rv = 0.130;
N_r = -1.9;
N_rr = -0.75;
N_rrr = 0 ;
N_vr = 0.080;

d11 = - X_u - X_uu  * abs(u) - X_uuu * u^2 ;
d22 = - Y_v - Y_vv  * abs(v) - Y_vvv * v^2 - Y_rv * abs(r) ;
d23 = - Y_r - Y_vr  * abs(v) - Y_rr * abs(r) - Y_rrr * r^2 ;
d32 = - N_v - N_vv  * abs(v) - N_vvv * v^2 - N_rv * abs(r) ;
d33 = - N_r - N_vr  * abs(v) - N_rr * abs(r) - N_rrr * r^2 ;

D = [ d11 , 0     ,   0          ;
      0  ,   d22  ,  d23         ;
      0  ,   d32  ,  d33       ] ;    % Damping matrix

 
%% TUNING & ALGORITHM
  
L1 = L1_o*eye(3) ;  % Diagonal Matrices are more simple for tuning
L2 = L2_o*eye(3) ;
L3 = L3_o*eye(3) ;
K2 = eye(3) ;       % See Appendix

R = [cos(psi),-sin(psi), 0;
     sin(psi), cos(psi), 0;
     0       ,   0     , 1 ] ;  % Rotation Matrix
 
 
A = [ L1            , R           , zeros(3)   ;
    Inv*K2*R'*L2 , -Inv*D   , Inv*R'  ;
    L3              , zeros(3)    , zeros(3)   ];   % State Space Matrix


Bu = [0;0;0;Inv*Tau;0;0;0]; % Control Input (vertical vector)


x_o = x + [eta_m(1)-2*x(1);
           eta_m(2)-2*x(2);
           eta_m(3)-2*x(3);
           0;0;0;  0;0;0 ]; % See Observer Design (vertical vector)

       
x_dot = A*x_o + Bu ;



end

== matlab function ctrl_student_HIL/DROP DETECTOR (CASE B)/DROP DETECTOR ==
  data: eta input; Mx0 input; My0 input; Drop output; Mx1 output; My1 output
function [Drop,Mx1,My1] = detectGPSDropOut(eta,Mx0,My0)

  x = eta(1);
  y = eta(2);
  
  Mx0 = Mx0';
  My0 = My0';
  
  Mx1 = [Mx0(2),Mx0(3),Mx0(4),Mx0(5),Mx0(6),Mx0(7),Mx0(8),Mx0(9),Mx0(10),x];
  My1 = [My0(2),My0(3),My0(4),My0(5),My0(6),My0(7),My0(8),My0(9),My0(10),y];
  
  if all(Mx1 - Mx0) && all(My1 - My0)
      Drop = 1;
  else
      Drop = 0;
  end
 

end

== matlab function ctrl_student_HIL/Noise generator/Downsample	signal/MATLAB Function ==
  data: f input; h input; i input; count output
function count = fcn(f,h,i)
%#codegen
sampling_time = 1/f;
if (i+1)*h >= sampling_time
    count = 0;
else
    count = i+1;
end

== matlab function ctrl_student_HIL/Noise generator/Sample & hold/MATLAB Function1 ==
  data: counter input; input input; hold input; output output
function output = fcn(counter,input,hold)
%#codegen

if counter == 0
    output = input;
else
    output = hold;
end

== matlab function ctrl_student_HIL/SWITCH ==
  data: eta1 input; eta0 input; Drop input; Eta output
function Eta = fcn(eta1,eta0,Drop)

if Drop == 1
    Eta = eta1;
else
    Eta = eta0;
end

%%Eta = [0,0,0]';

end

== matlab function ctrl_student_HIL/Tank (CASE B)/TANK LIMITS (CASE B)/Tank Limits ==
  data: x_d1 output; x_d input; eta input; M1 output; M input; s1 output; s input

function [x_d1,M1,s1] = reverseIfOutOfBounds(x_d, eta, M,s)
      
  x = eta(1);
  y = eta(2);
  %psi = eta(3);

  K = 2;
  minX = -3/K;
  maxX = 3/K;
  minY = -5/K;
  maxY = 5/K;
  
  
  % If too close from edges, change sign
  if M == 0
    if (x < minX) || (x > maxX) || (y < minY) || (y > maxY)
        s1 = - s;
        M1 = 1;
    else
        M1=M;
        s1=s;
    end
  else % M = 1
      if (x >= minX/2) && (x <= maxX/2) && (y >= minY/2) && (y <= maxY/2)
        M1 = 0;
        s1=s;
    else
        M1=M;
        s1=s;
      end
  end
  
  x_d1 =s1*x_d;
  
end

== matlab function ctrl_student_HIL/joystick/Bow thruster ==
  data: u_BT output; L2 input; R2 input
function u_BT  = fcn(L2,R2)
%#codegen

u_BT = (R2-L2)/2 ;

end

== matlab function ctrl_student_HIL/joystick/MATLAB Function ==
  data: u output; a output; PosX input; PosY input
function [u,a] = fcn(PosX,PosY)
%#codegen

a = atan2(PosX,-PosY);
u = min(1,sqrt(PosX^2+PosY^2));
end

== matlab function ctrl_student_HIL/joystick/MATLAB Function1 ==
  data: u_VSP output; a_VSP output; PosX input; PosY input
function [u_VSP,a_VSP] = fcn(PosX,PosY)
%#codegen
%The force angle.
a_VSP = atan2(PosX,-PosY);
%generalised force
u_VSP = min(1,sqrt(PosX^2+PosY^2));
end

== matlab function ctrl_student_HIL/joystick/Voith Schneider Propeller ==
  data: Omega1 output; Omega2 output; ArrowUp input; ArrowDown input; t input; Omega0 input
function [Omega1,Omega2] = fcn(ArrowUp,ArrowDown,t,Omega0)
%#codegen
%find the remain time.
b = mod(t,1);
%use if sentence to calculate the correct rotational speed.
if  b <= 0.01
    Omega = Omega0 + 0.1*ArrowUp - 0.1*ArrowDown;
else
    Omega = Omega0;
end


%define the value of rotational speed.
Omega1 = Omega;
Omega2 = Omega;

end
